simulink model "LinearSys"  (Simulink 8.0)
settings: Solver=ode45  StartTime=0.0  StopTime=10  MaxStep=0.1  RelTol=1e-3
values from neighbouring files (symbols this model uses):
  Ac = [sum(Ay), sum(Ath), sum(Aph) ... (first row only)    [simpleSys.m]
  As = [0,            1, 0,             0, 0,             0, 0 ... (first row only)    [simpleSys.m]
  Bs = [zeros(1,8) ... (first row only)    [simpleSys.m]
  Cs = [1, 0, 0, 0, 0, 0, 0 ... (first row only)    [simpleSys.m]
  Ds = zeros(3,8)    [simpleSys.m]
  Filter_Coef = 1000    [SimParam.m]    (also in simpleSys.m)
  Gc = [sum(G) - mass*g ; Lx'*G ; Lz'*G]    [simpleSys.m]
  M = [mass 0 0; 0 Ix 0 ; 0 0 Iz]    [simpleSys.m]
  nullProj = eye(8) - pinvBc*Bc    [simpleSys.m]
  pinvBc = pinv(Bc)    [simpleSys.m]
  w = 60    [simpleSys.m]
  x0 = [y0; 0; theta0; 0; phi0; 0; 1]    [simpleSys.m]
  xdes = [y, theta, phi]    [simpleSys.m]
undefined symbols (not defined in the file): K_d, K_i, K_p, phi0, theta0, y0
libraries: dspstat3 x6
settings Model: Creator=nitisht  LastModifiedBy=nitisht  SimulationMode=accelerator
settings HardwareCC: ProdBitPerLong=64  ProdBitPerPointer=64  ProdWordSize=64  ProdHWDeviceType=Intel->x86-64
settings RTWCC: RTWCompilerOptimization=On

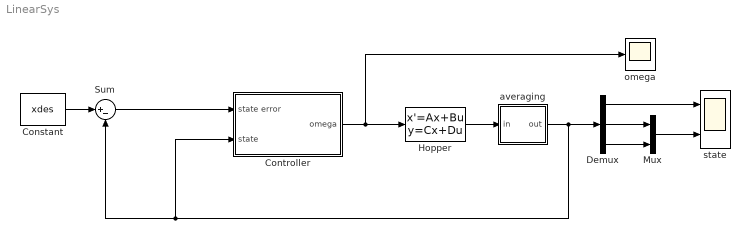
== system LinearSys ==
  Constant : Constant  Value=xdes
  Controller : Subsystem
  Demux : Demux  Outputs=3
  Hopper : StateSpace  A=As  B=Bs  C=Cs  D=Ds  X0=x0
  Mux : Mux  Inputs=2
  Sum : Sum  Inputs=|+-
  averaging : Subsystem  mask{T_win=2*pi/w, x_init=[y0, theta0, phi0]}
      mask prompts: T_win "window (s)"; x_init "Initial condition"
  omega : Scope
      settings: TimeRange=600  YMin=42.5  YMax=70
  state : Scope  NumInputPorts=2
      settings: TimeRange=600  YMin=0.015~0  YMax=0.015~7.5
  wires:
  Hopper/1 -> averaging/1(in)
  Constant/1 -> Sum/1
  averaging/1(out) -> Controller/2(state), Sum/2, Demux/1
  Controller/1(omega) -> omega/1, Hopper/1
  Sum/1 -> Controller/1(state error)
  Demux/1 -> state/1
  Demux/2 -> Mux/1
  Demux/3 -> Mux/2
  Mux/1 -> state/2

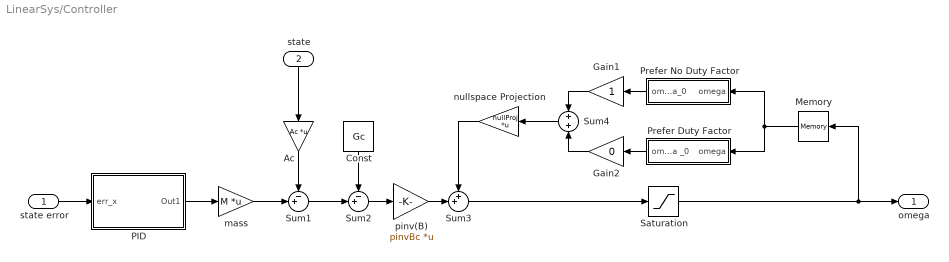
== system LinearSys/Controller ==
  state error : Inport
  state : Inport  Port=2
  Ac : Gain  Gain=Ac  Multiplication=Matrix(K*u)
  Const : Constant  Value=Gc
  Gain1 : Gain
  Gain2 : Gain  Gain=0
  Memory : Memory  X0=w*ones(8,1)
  PID : Subsystem  mask{P=K_p, I=K_i, D=K_d, N=Filter_Coef}
      mask prompts: P "Proportional Gain"; I "Integral Gain"; D "Derivative Gain"; N "Filter Coefficient"
  Prefer Duty Factor : Subsystem
  Prefer No Duty Factor : Subsystem
  Saturation : Saturate  UpperLimit=100  LowerLimit=10
  Sum1 : Sum  Inputs=-+|
  Sum2 : Sum  Inputs=-+|
  Sum3 : Sum  Inputs=++|
  Sum4 : Sum  Inputs=+|+
  mass : Gain  Gain=M  Multiplication=Matrix(K*u)
  nullspace Projection : Gain  Gain=nullProj  Multiplication=Matrix(K*u)
  pinv(B) : Gain  Gain=pinvBc  Multiplication=Matrix(K*u)
  omega : Outport
  wires:
  Gain2/1 -> Sum4/2
  state/1 -> Ac/1
  Sum2/1 -> pinv(B)/1
  mass/1 -> Sum1/2
  Memory/1 -> Prefer Duty Factor/1(omega), Prefer No Duty Factor/1(omega)
  Prefer No Duty Factor/1(omega_0) -> Gain1/1
  Prefer Duty Factor/1(omega _0) -> Gain2/1
  Gain1/1 -> Sum4/1
  state error/1 -> PID/1(err_x)
  Sum3/1 -> Saturation/1
  Sum4/1 -> nullspace Projection/1
  PID/1(Out1) -> mass/1
  Saturation/1 -> Memory/1, omega/1
  Ac/1 -> Sum1/1
  pinv(B)/1 -> Sum3/2
  nullspace Projection/1 -> Sum3/1
  Sum1/1 -> Sum2/2
  Const/1 -> Sum2/1

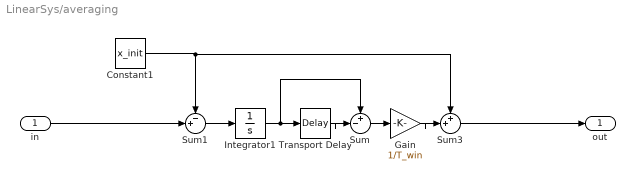
== system LinearSys/averaging ==
  in : Inport
  Constant1 : Constant  Value=x_init
  Gain : Gain  Gain=1/T_win
  Integrator1 : Integrator
  Sum : Sum  Inputs=+-|
  Sum1 : Sum  Inputs=-+|
  Sum3 : Sum  Inputs=++|
  Transport Delay : TransportDelay  DelayTime=T_win
  out : Outport
  wires:
  Sum/1 -> Gain/1
  Sum3/1 -> out/1
  Integrator1/1 -> Transport Delay/1, Sum/1
  Transport Delay/1 -> Sum/2
  Sum1/1 -> Integrator1/1
  Constant1/1 -> Sum1/1, Sum3/1
  Gain/1 -> Sum3/2
  in/1 -> Sum1/2

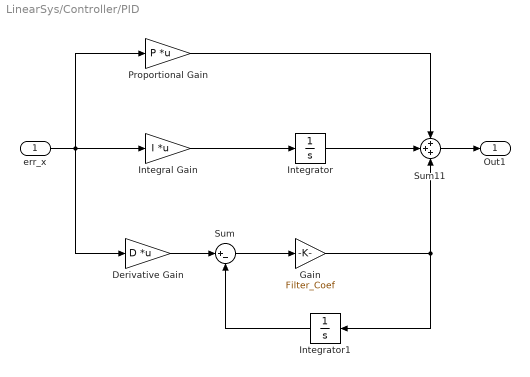
== system LinearSys/Controller/PID ==
  err_x : Inport
  Derivative Gain : Gain  Gain=D  Multiplication=Matrix(K*u)
  Gain : Gain  Gain=Filter_Coef
  Integral Gain : Gain  DisableCoverage=on  Gain=I  Multiplication=Matrix(K*u)
  Integrator : Integrator
  Integrator1 : Integrator
  Proportional Gain : Gain  Gain=P  Multiplication=Matrix(K*u)
  Sum : Sum  Inputs=|+-
  Sum11 : Sum  Inputs=+++
  Out1 : Outport
  wires:
  Proportional Gain/1 -> Sum11/1
  Sum11/1 -> Out1/1
  Integrator/1 -> Sum11/2
  Gain/1 -> Integrator1/1, Sum11/3
  err_x/1 -> Derivative Gain/1, Integral Gain/1, Proportional Gain/1
  Derivative Gain/1 -> Sum/1
  Sum/1 -> Gain/1
  Integrator1/1 -> Sum/2
  Integral Gain/1 -> Integrator/1

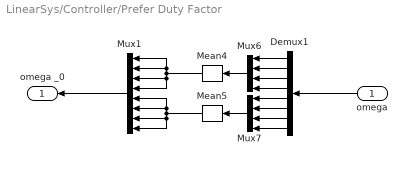
== system LinearSys/Controller/Prefer Duty Factor ==
  omega : Inport
  Demux1 : Demux  Outputs=8
  Mean4 : dspstat3/Mean  run=off  reset_popup=None  InputProcessing=Columns as channels (frame based)  directionMode=Each column  dimension=1  treatSBRowAsCol=on  roiEnable=off  roiType=Rectangles  roiPortion=Entire ROI  roiOutput=Individual statistics for each ROI  roiFlag=off  outputDataTypeStr=Inherit: Same as accumulator  outputLastDataTypeStr=Inherit: Same as accumulator  outputMin=[]  outputMax=[]  roundingMode=Floor  overflowMode=off
  Mean5 : dspstat3/Mean  run=off  reset_popup=None  InputProcessing=Columns as channels (frame based)  directionMode=Each column  dimension=1  treatSBRowAsCol=on  roiEnable=off  roiType=Rectangles  roiPortion=Entire ROI  roiOutput=Individual statistics for each ROI  roiFlag=off  outputDataTypeStr=Inherit: Same as accumulator  outputLastDataTypeStr=Inherit: Same as accumulator  outputMin=[]  outputMax=[]  roundingMode=Floor  overflowMode=off
  Mux1 : Mux  Inputs=8
  Mux6 : Mux
  Mux7 : Mux
  omega _0 : Outport
  wires:
  Mean4/1 -> Mux1/3, Mux1/4, Mux1/1, Mux1/2
  Demux1/6 -> Mux7/2
  Demux1/3 -> Mux6/3
  Demux1/5 -> Mux7/1
  Mux1/1 -> omega _0/1
  Demux1/8 -> Mux7/4
  Demux1/1 -> Mux6/1
  Demux1/7 -> Mux7/3
  Demux1/4 -> Mux6/4
  omega/1 -> Demux1/1
  Mean5/1 -> Mux1/7, Mux1/8, Mux1/5, Mux1/6
  Mux7/1 -> Mean5/1
  Mux6/1 -> Mean4/1
  Demux1/2 -> Mux6/2

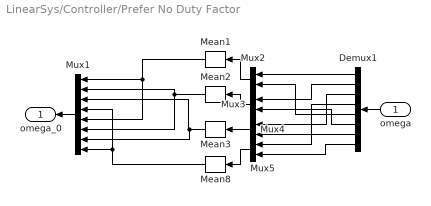
== system LinearSys/Controller/Prefer No Duty Factor ==
  omega : Inport
  Demux1 : Demux  Outputs=8
  Mean{1..3,8} (4 alike) : dspstat3/Mean  run=off  reset_popup=None  InputProcessing=Columns as channels (frame based)  directionMode=Each column  dimension=1  treatSBRowAsCol=on  roiEnable=off  roiType=Rectangles  roiPortion=Entire ROI  roiOutput=Individual statistics for each ROI  roiFlag=off  outputDataTypeStr=Inherit: Same as accumulator  outputLastDataTypeStr=Inherit: Same as accumulator  outputMin=[]  outputMax=[]  roundingMode=Floor  overflowMode=off
  Mux1 : Mux  Inputs=8
  Mux{2..5} (4 alike) : Mux  Inputs=2
  omega_0 : Outport
  wires:
  Demux1/7 -> Mux4/2
  Demux1/1 -> Mux2/1
  Demux1/6 -> Mux3/2
  Mux2/1 -> Mean1/1
  Mux4/1 -> Mean3/1
  Mux3/1 -> Mean2/1
  Demux1/2 -> Mux3/1
  Mean3/1 -> Mux1/7, Mux1/3
  Demux1/5 -> Mux2/2
  Mux1/1 -> omega_0/1
  Mean1/1 -> Mux1/5, Mux1/1
  omega/1 -> Demux1/1
  Mean2/1 -> Mux1/6, Mux1/2
  Demux1/3 -> Mux4/1
  Demux1/4 -> Mux5/1
  Mean8/1 -> Mux1/8, Mux1/4
  Demux1/8 -> Mux5/2
  Mux5/1 -> Mean8/1
